simulink model "lab04es01a_schema"  (R2021b)
settings: Solver=VariableStepAuto  StartTime=0.0  StopTime=20  RelTol=1e-3
values from neighbouring files (symbols this model uses):
  beta = 14e-6    (= 1.4e-05)    [L_21_04_21.m]    (also in L_21_04_27_Simulink.m; L_27_04_21_Simulink.m; Lezione_21_04_21.m)
  Km = 0.05335    [L_21_04_21.m]    (also in L_21_04_27_Simulink.m; L_27_04_21_Simulink.m; Lezione_21_04_21.m)
  Ra = 6    [L_21_04_21.m]    (also in L_21_04_27_Simulink.m; L_27_04_21_Simulink.m; Lezione_21_04_21.m)
undefined symbols (not defined in the file or in its folder): Ka
libraries: cstblocks x2
settings Model: Creator=francescafornasier  LastModifiedBy=francescafornasier

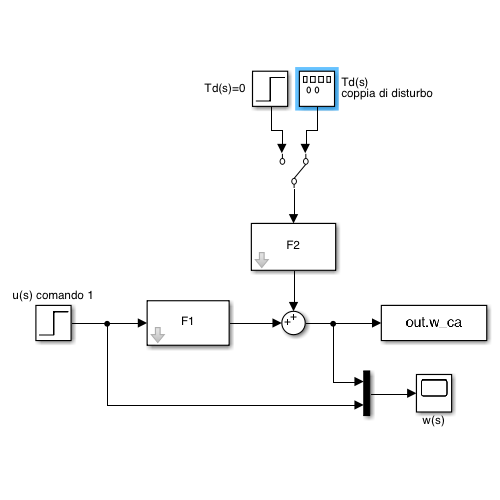
[thumbnail: Simulink's stored preview of the top-level diagram]
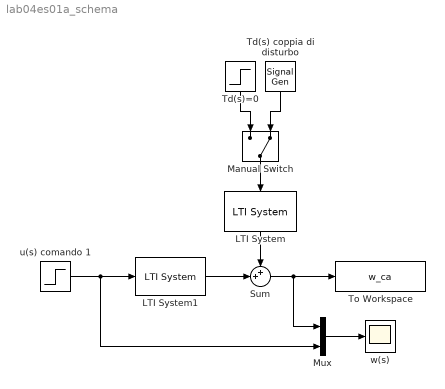
== system lab04es01a_schema ==
  LTI System : cstblocks/LTI System  sys=F2  IC=[]
  LTI System1 : cstblocks/LTI System  sys=F1  IC=[]
  Manual Switch : ManualSwitch  CurrentSetting=0
  Mux : Mux  Inputs=2
  Sum : Sum  Inputs=++|
  Td(s) coppia di disturbo : SignalGenerator  WaveForm=square  Amplitude=0.05  Frequency=0.1
  Td(s)=0 : Step  Time=0  After=0  SampleTime=0
  To Workspace : ToWorkspace  VariableName=w_ca  SaveFormat=Timeseries  SampleTime=-1
  u(s) comando 1 : Step  Time=0  After=((Ka*Km)/(beta*Ra+Km^2))^(-1)  SampleTime=0
  w(s) : Scope
  wires:
  LTI System1/1 -> Sum/2
  LTI System/1 -> Sum/1
  Sum/1 -> Mux/1, To Workspace/1
  Mux/1 -> w(s)/1
  u(s) comando 1/1 -> Mux/2, LTI System1/1
  Manual Switch/1 -> LTI System/1
  Td(s) coppia di disturbo/1 -> Manual Switch/2
  Td(s)=0/1 -> Manual Switch/1
